simulink model "PATH_FOLLOWING_2018"  (R2018b)
settings: Solver=VariableStepAuto  StartTime=0  StopTime=T  MaxStep=0.1  RelTol=1e-3
values from neighbouring files (symbols this model uses):
  N = 5000    [PATH_PLANNING.m]
  x = R*cos(t)+Xc    [PATH_PLANNING.m]    (also in path_points.m = a*((q-1)*cos(u)+ k*cos((q-1)*u)) - a*(q-1+k))
  y = R*sin(t)+Yc    [PATH_PLANNING.m]    (also in path_points.m = a*((q-1)*sin(u)- k*sin((q-1)*u)))
  z = -13*ones(sz,1)    [PATH_PLANNING.m]    (also in path_points.m = b*sin(0.5*q*u) - 10)
undefined symbols (not defined in the file or in its folder): sigbuilder_block, X, Y, Z
libraries: sm_lib x29, nesl_utility x13, simulink x6
(part 2 of 2)

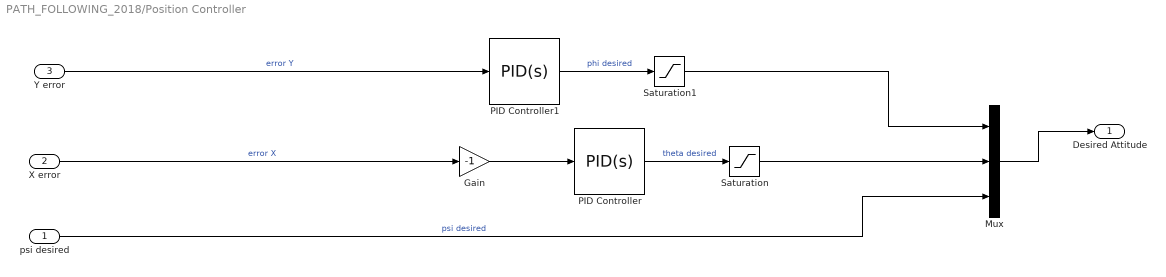
== system PATH_FOLLOWING_2018/Position Controller ==
  psi desired : Inport
  X error : Inport  Port=2
  Y error : Inport  Port=3
  Gain : Gain  Gain=-1
  Mux : Mux  Inputs=3
  PID Controller : simulink/Continuous/PID Controller  Controller=PID  Form=Parallel  TimeDomain=Continuous-time  SampleTime=-1  IntegratorMethod=Forward Euler  ControllerParametersSource=internal  P=0.1  I=0.001  D=0.2  UseFilter=on  N=100  TunerSelectOption=Transfer Function Based (PID Tuner App)  InitialConditionSource=internal  InitialConditionForIntegrator=0  InitialConditionForFilter=0  DifferentiatorICPrevScaledInput=0  ExternalReset=none  TrackingMode=off  Kt=1  LimitOutput=off  UpperSaturationLimit=inf  LowerSaturationLimit=-inf  LinearizeAsGain=on  AntiWindupMode=none  Kb=1  POutMin=[]  POutMax=[]  IOutMin=[]  IOutMax=[]  DOutMin=[]  DOutMax=[]  NOutMin=[]  NOutMax=[]  SumOutMin=[]  SumOutMax=[]  SaturationOutMin=[]  SaturationOutMax=[]  PParamMin=[]  PParamMax=[]  IParamMin=[]  IParamMax=[]  DParamMin=[]  DParamMax=[]  NParamMin=[]  NParamMax=[]  KbParamMin=[]  KbParamMax=[]  KtParamMin=[]  KtParamMax=[]  KbOutMin=[]  KbOutMax=[]  KtOutMin=[]  KtOutMax=[]  IntegratorOutMin=[]  IntegratorOutMax=[]  FilterOutMin=[]  FilterOutMax=[]  SumI1OutMin=[]  SumI1OutMax=[]  SumI2OutMin=[]  SumI2OutMax=[]  SumI3OutMin=[]  SumI3OutMax=[]  SumI4OutMin=[]  SumI4OutMax=[]  SumDOutMin=[]  SumDOutMax=[]  DifferentiatorOutMin=[]  DifferentiatorOutMax=[]  FilterDiffOutCoefMin=[]  FilterDiffOutCoefMax=[]  ReciprocalOutMin=[]  ReciprocalOutMax=[]  SumDenOutMin=[]  SumDenOutMax=[]  SumNumOutMin=[]  SumNumOutMax=[]  DivideOutMin=[]  DivideOutMax=[]  IntegratorContinuousStateAttributes=''  IntegratorStateMustResolveToSignalObject=off  IntegratorRTWStateStorageClass=Auto  FilterContinuousStateAttributes=''  FilterStateMustResolveToSignalObject=off  FilterRTWStateStorageClass=Auto  ParallelPVariant=InternalParameters  IdealPVariant=Disabled  IVariant=InternalParameters  DVariant=InternalParameters  IntegratorVariant=Continuous  SatVariant=Disabled  AWVariant=Passthrough  PCopyVariant=Disabled  TRVariant=Disabled  FdbkBlocksVariant=Forward  IdealPFdbkVariant=Disabled  SatFdbkVariant=Disabled  DerivativeFilterVariant=ContFilter  NVariant=InternalParameters  NCopyVariant=Disabled  FilterICVariant=InternalICsFilter  IntegratorICVariant=InternalICs  ExternalResetVariant=Disabled  TRSumVariant=Passthrough  SumFdbkVariant=Disabled  SumVariant=Sum_PID
  PID Controller1 : simulink/Continuous/PID Controller  Controller=PID  Form=Parallel  TimeDomain=Continuous-time  SampleTime=-1  IntegratorMethod=Forward Euler  ControllerParametersSource=internal  P=0.1  I=0.001  D=0.2  UseFilter=on  N=100  TunerSelectOption=Transfer Function Based (PID Tuner App)  InitialConditionSource=internal  InitialConditionForIntegrator=0  InitialConditionForFilter=0  DifferentiatorICPrevScaledInput=0  ExternalReset=none  TrackingMode=off  Kt=1  LimitOutput=off  UpperSaturationLimit=inf  LowerSaturationLimit=-inf  LinearizeAsGain=on  AntiWindupMode=none  Kb=1  POutMin=[]  POutMax=[]  IOutMin=[]  IOutMax=[]  DOutMin=[]  DOutMax=[]  NOutMin=[]  NOutMax=[]  SumOutMin=[]  SumOutMax=[]  SaturationOutMin=[]  SaturationOutMax=[]  PParamMin=[]  PParamMax=[]  IParamMin=[]  IParamMax=[]  DParamMin=[]  DParamMax=[]  NParamMin=[]  NParamMax=[]  KbParamMin=[]  KbParamMax=[]  KtParamMin=[]  KtParamMax=[]  KbOutMin=[]  KbOutMax=[]  KtOutMin=[]  KtOutMax=[]  IntegratorOutMin=[]  IntegratorOutMax=[]  FilterOutMin=[]  FilterOutMax=[]  SumI1OutMin=[]  SumI1OutMax=[]  SumI2OutMin=[]  SumI2OutMax=[]  SumI3OutMin=[]  SumI3OutMax=[]  SumI4OutMin=[]  SumI4OutMax=[]  SumDOutMin=[]  SumDOutMax=[]  DifferentiatorOutMin=[]  DifferentiatorOutMax=[]  FilterDiffOutCoefMin=[]  FilterDiffOutCoefMax=[]  ReciprocalOutMin=[]  ReciprocalOutMax=[]  SumDenOutMin=[]  SumDenOutMax=[]  SumNumOutMin=[]  SumNumOutMax=[]  DivideOutMin=[]  DivideOutMax=[]  IntegratorContinuousStateAttributes=''  IntegratorStateMustResolveToSignalObject=off  IntegratorRTWStateStorageClass=Auto  FilterContinuousStateAttributes=''  FilterStateMustResolveToSignalObject=off  FilterRTWStateStorageClass=Auto  ParallelPVariant=InternalParameters  IdealPVariant=Disabled  IVariant=InternalParameters  DVariant=InternalParameters  IntegratorVariant=Continuous  SatVariant=Disabled  AWVariant=Passthrough  PCopyVariant=Disabled  TRVariant=Disabled  FdbkBlocksVariant=Forward  IdealPFdbkVariant=Disabled  SatFdbkVariant=Disabled  DerivativeFilterVariant=ContFilter  NVariant=InternalParameters  NCopyVariant=Disabled  FilterICVariant=InternalICsFilter  IntegratorICVariant=InternalICs  ExternalResetVariant=Disabled  TRSumVariant=Passthrough  SumFdbkVariant=Disabled  SumVariant=Sum_PID
  Saturation : Saturate  UpperLimit=0.7  LowerLimit=-0.7
  Saturation1 : Saturate  UpperLimit=0.7  LowerLimit=-0.7
  Desired Attitude : Outport  PortDimensions=3
  wires:
  Y error/1 -> PID Controller1/1  "error Y"
  Mux/1 -> Desired Attitude/1
  PID Controller1/1 -> Saturation1/1  "phi desired"
  PID Controller/1 -> Saturation/1  "theta desired"
  X error/1 -> Gain/1  "error X"
  Gain/1 -> PID Controller/1
  Saturation/1 -> Mux/2
  Saturation1/1 -> Mux/1
  psi desired/1 -> Mux/3  "psi desired"

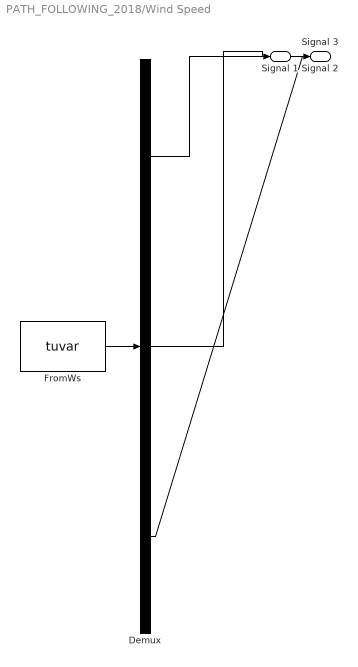
== system PATH_FOLLOWING_2018/Wind Speed ==
  Demux : Demux  Tag=STV Demux  Outputs=3
      settings: DisplayOption=none
  FromWs : FromWorkspace  Tag=STV FromWs  VariableName=tuvar
      SigBuilderData=|
      | common.afterFinalStr = 'Extrapolate'
      | common.sampleTime = 0
      | dataSet.timeRange = [0 10]
      | dataSet.name = 'Group 1'
      | sbobj.Groups.Name = 'Group 1'
      | sbobj.Groups.Signals(1).Name = 'Signal 1'
      | sbobj.Groups.Signals(1).XData = [0 4 4 7 7 10]
      | sbobj.Groups.Signals(1).YData = [0 0.01 1.15 1.15 0 0]
      | sbobj.Groups.Signals(2).Name = 'Signal 2'
      | sbobj.Groups.Signals(2).XData = [0 3.5 4 6 7 10]
      | sbobj.Groups.Signals(2).YData = [0 0 1 1 0 0]
      | sbobj.Groups.Signals(3).Name = 'Signal 3'
      | sbobj.Groups.Signals(3).XData = [0 3 4 6 6 10]
      | sbobj.Groups.Signals(3).YData = [0 0 0.14 0.14 0 0]
  Signal 1 : Outport  Tag=STV Outport
  Signal 2 : Outport  Tag=STV Outport  Port=2
  Signal 3 : Outport  Tag=STV Outport  Port=3
  wires:
  Demux/1 -> Signal 1/1
  FromWs/1 -> Demux/1
  Demux/2 -> Signal 2/1
  Demux/3 -> Signal 3/1

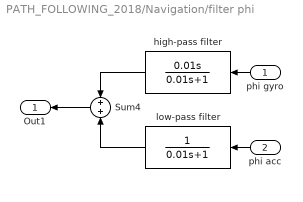
== system PATH_FOLLOWING_2018/Navigation/filter phi ==
  phi gyro : Inport
  phi acc : Inport  Port=2
  Sum4 : Sum  Inputs=+|+
  high-pass filter : TransferFcn  Numerator=[0.01 0]  Denominator=[0.01 1]
  low-pass filter : TransferFcn  Denominator=[0.01 1]
  Out1 : Outport
  wires:
  high-pass filter/1 -> Sum4/1
  phi gyro/1 -> high-pass filter/1
  phi acc/1 -> low-pass filter/1
  low-pass filter/1 -> Sum4/2
  Sum4/1 -> Out1/1

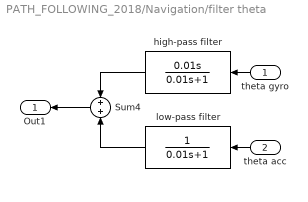
== system PATH_FOLLOWING_2018/Navigation/filter theta ==
  theta gyro : Inport
  theta acc : Inport  Port=2
  Sum4 : Sum  Inputs=+|+
  high-pass filter : TransferFcn  Numerator=[0.01 0]  Denominator=[0.01 1]
  low-pass filter : TransferFcn  Denominator=[0.01 1]
  Out1 : Outport
  wires:
  Sum4/1 -> Out1/1
  low-pass filter/1 -> Sum4/2
  theta acc/1 -> low-pass filter/1
  theta gyro/1 -> high-pass filter/1
  high-pass filter/1 -> Sum4/1

== matlab function PATH_FOLLOWING_2018/Wind ==
  data: V_wind input; Fw output; V input
function Fw = fcn(V_wind,V)
CD = 0.20 ;
A_side = 1.6 * 0.6;

Fw = 0.5*A_side*CD*(V_wind-V).*abs(V_wind-V);

== matlab function PATH_FOLLOWING_2018/Plant ==
  data: phi_ output; theta_ output; psi_ output; phi output; theta output; psi output; X_dd output; w1 input; w2 input; w3 input; w4 input; q0 input; q1 input; q2 input; q3 input; w_d output; w input; q0_d output; q1_d output; q2_d output; q3_d output; F_wind input
function [phi_,theta_,psi_,phi,theta,psi,X_dd,w_d,q0_d,q1_d,q2_d,q3_d]= fcn( w1, w2, w3, w4, q0, q1,  q2, q3, w, F_wind)
m = 10.073;
g = 9.81;
CT = 3.42e-4;
Cm = 7.76e-6;
b = 0.6;
gama1 = 0;
gama2 = 0;

T1 = 0.5*CT*w1^2;
T2 = 0.5*CT*w2^2;
T3 = 0.5*CT*w3^2;
T4 = 0.5*CT*w4^2;


R_I_b = [ q0^2+q1^2-q2^2-q3^2 , 2*(q1*q2 + q0*q3), 2*(q1*q3-q0*q2);
       2*(q1*q2-q0*q3), q0^2-q1^2+q2^2-q3^2 , 2*(q2*q3+q0*q1);
       2*(q1*q3+q0*q2) , 2*(q2*q3-q0*q1), q0^2-q1^2-q2^2+q3^2 ];
   
R_b_I = R_I_b';
F = R_b_I * [T1*sin(gama1)+T2*sin(gama2);0;-(T1*cos(gama1)+T2*cos(gama2)+T3+T4)];

X_dd = (F+[0;0;m*g]+F_wind)/m ;

I = [ 0.09696    -0.000007  0.0163;
      -0.000007     0.161      0.0 ;
     0.0163   0.0  0.210 ];
 
p = w(1); q = w(2); r = w(3);

Sw = [0 -r  q;...
      r  0 -p;...
     -q  p  0];

M = [b*( -T1*cos(gama1)+T2*cos(gama2)+T3-T4 ) + Cm/CT*( -T1*sin(gama1)+T2*sin(gama2) );...
     b*( T1*cos(gama1)+T2*cos(gama2)-T3-T4 );...
     Cm/CT *( T1*cos(gama1)-T2*cos(gama2)+T3-T4 ) + b*T2*sin(gama2) - b*T1*sin(gama1)];
 
w_d = I\(M - Sw*I*w);

G=0.5*[0 -p -q -r;
       p  0  r -q;
       q -r  0  p;
       r  q -p  0];
   
q_d = G*[q0;q1;q2;q3];
q0_d=q_d(1);
q1_d=q_d(2);
q2_d=q_d(3);
q3_d=q_d(4);

phi=atan(2*(q0*q1+q2*q3)/(1-2*(q1^2+q2^2)));
theta=real(asin(complex(2*(q0*q2-q1*q3))));
psi=atan2(2*(q0*q3+q1*q2),(1-2*(q2^2+q3^2)));
angles = quat2eul([q0,q1,q2,q3],'XYZ');
phi_=angles(1); theta_=angles(2); psi_=angles(3);
%phi_=0; theta_=0; psi_=0;
end

== matlab function PATH_FOLLOWING_2018/Mixer ==
  data: Mx input; w1 output; w2 output; My input; Mz input; w3 output; w4 output; fz input
function [w1,w2,w3,w4] = fcn(Mx,My,Mz,fz)
% both M and f should be in body's coordinate
m = 10.073;
g = 9.81;
CT = 3.42e-4;
Cm = 7.76e-6;
b = 0.6;
gama1=0; gama2=0;

c1=cos(gama1); c2=cos(gama2); s1=sin(gama1); s2=sin(gama2);
AB =[-b*c1-Cm/CT*s1, b*c2+Cm/CT*s2,    b,   -b;
    b*c1,          b*c2,             -b,      -b;
    -b*s1+Cm/CT*c1, b*s2-Cm/CT*c2,     Cm/CT,  -Cm/CT;
     -c1,          -c2,               -1,      -1];

T = AB\[Mx;My;Mz;fz];
T1=T(1);  T2=T(2);  T3=T(3);  T4=T(4);  

w1 = sqrt(T1/(0.5*CT));
w2 = sqrt(T2/(0.5*CT));
w3 = sqrt(T3/(0.5*CT));
w4 = sqrt(T4/(0.5*CT));
end

== matlab function PATH_FOLLOWING_2018/Inertia to body transformer ==
  data: input input; y output; phi input; theta input; psi input
function y = fcn(input,phi,theta,psi)
phi=0; theta=0;
xI=input(1); yI=input(2); zI=input(3); 
XI=[xI;yI;zI];
y = zeros(3,1);

R_I_b = [cos(psi)*cos(theta), sin(psi)*cos(theta), -sin(theta);...
     -sin(psi)*cos(phi)+cos(psi)*sin(theta)*sin(phi), cos(psi)*cos(phi)+sin(psi)*sin(theta)*sin(phi), cos(theta)*sin(phi);...
     sin(psi)*sin(phi)+cos(psi)*sin(theta)*cos(phi), -cos(psi)*sin(phi)+sin(psi)*sin(theta)*cos(phi), cos(theta)*cos(phi)];

Xb = R_I_b*XI;

y = [ Xb(1); Xb(2); Xb(3)];
end

== matlab function PATH_FOLLOWING_2018/Attitude Controller/wrapping to pi ==
  data: psi_error input; y output
function y = fcn(psi_error)
y = wrapToPi(psi_error);

== matlab function PATH_FOLLOWING_2018/Navigation/angular velocity to euler rate ==
  data: euler input; euler_rate output; ang_vel input
function euler_rate = fcn(euler,ang_vel)
euler_rate = zeros(3,1);
phi = euler(1); theta = euler(2); psi = euler(3);
euler_rate =[1 sin(phi)*tan(theta) cos(phi)*tan(theta);
    0 cos(phi) -sin(phi);
    0 sin(phi)/cos(theta) cos(phi)/cos(theta)] * [ang_vel(1);ang_vel(2);ang_vel(3)];
end

== matlab function PATH_FOLLOWING_2018/Navigation/body to inertia transform ==
  data: input input; y output; attitude input
function y = fcn(input,attitude)
xI=input(1); yI=input(2); zI=input(3); 
phi = attitude(1); theta = attitude(2); psi = attitude(3);
XI=[xI;yI;zI];

R_I_b = [cos(psi)*cos(theta), sin(psi)*cos(theta), -sin(theta);...
     -sin(psi)*cos(phi)+cos(psi)*sin(theta)*sin(phi), cos(psi)*cos(phi)+sin(psi)*sin(theta)*sin(phi), cos(theta)*sin(phi);...
     sin(psi)*sin(phi)+cos(psi)*sin(theta)*cos(phi), -cos(psi)*sin(phi)+sin(psi)*sin(theta)*cos(phi), cos(theta)*cos(phi)];

Xb = R_I_b'*XI;

y = [ Xb(1); Xb(2); Xb(3)];
end

== matlab function PATH_FOLLOWING_2018/Inertia to body transformer1 ==
  data: input input; y output; attitude input
function y = fcn(input,attitude)
xI=input(1); yI=input(2); zI=input(3); 
phi = attitude(1); theta = attitude(2); psi = attitude(3);
XI=[xI;yI;zI];

R_I_b = [cos(psi)*cos(theta), sin(psi)*cos(theta), -sin(theta);...
     -sin(psi)*cos(phi)+cos(psi)*sin(theta)*sin(phi), cos(psi)*cos(phi)+sin(psi)*sin(theta)*sin(phi), cos(theta)*sin(phi);...
     sin(psi)*sin(phi)+cos(psi)*sin(theta)*cos(phi), -cos(psi)*sin(phi)+sin(psi)*sin(theta)*cos(phi), cos(theta)*cos(phi)];

Xb = R_I_b*XI;

y = [ Xb(1); Xb(2); Xb(3)];
end

== matlab function PATH_FOLLOWING_2018/Navigation/accelerometer-estimated angles ==
  data: a input; phi output; theta output
function [phi,theta] = fcn(a)
g = 9.81;
theta = asin(clip(-a(1)/g));
phi = asin(clip(a(2)/(g*cos(theta))));
end

function out = clip(x)
lim = 1;
if x>abs(lim)
    out = abs(lim);
elseif  x<=abs(lim) && x>= -abs(lim)
    out = x;
else
    out = -abs(lim);
end

end
